simulink model "Falownik_2_4"  (R2023b)
settings: Solver=VariableStepAuto  StartTime=0.0  StopTime=50e-3  FixedStep=1e-9  RelTol=1e-3
libraries: spsSeriesRLCBranchLib x6, spsMosfetLib x4, simulink x2, spsCurrentMeasurementLib x2, spsOnDelayLib x2, spsVoltageMeasurementLib x2, spsDCVoltageSourceLib x1, spsRMSLib x1, spspowerguiLib x1
settings Model: Creator=szymo  LastModifiedBy=rolni
settings OptimizationCC: ReuseModelBlockBuffer=off
settings ModelReferenceCC: EnableRefExpFcnMdlSchedulingChecks=on

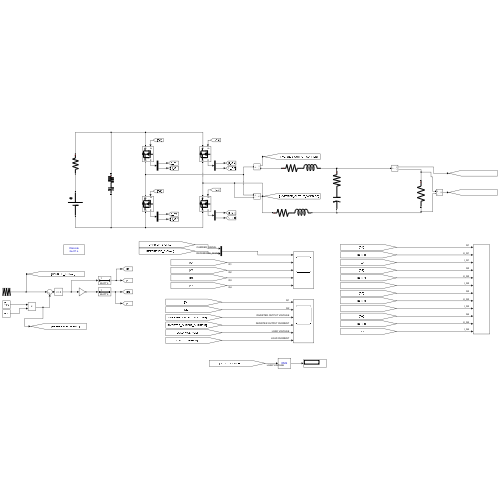
[thumbnail: Simulink's stored preview of the top-level diagram]
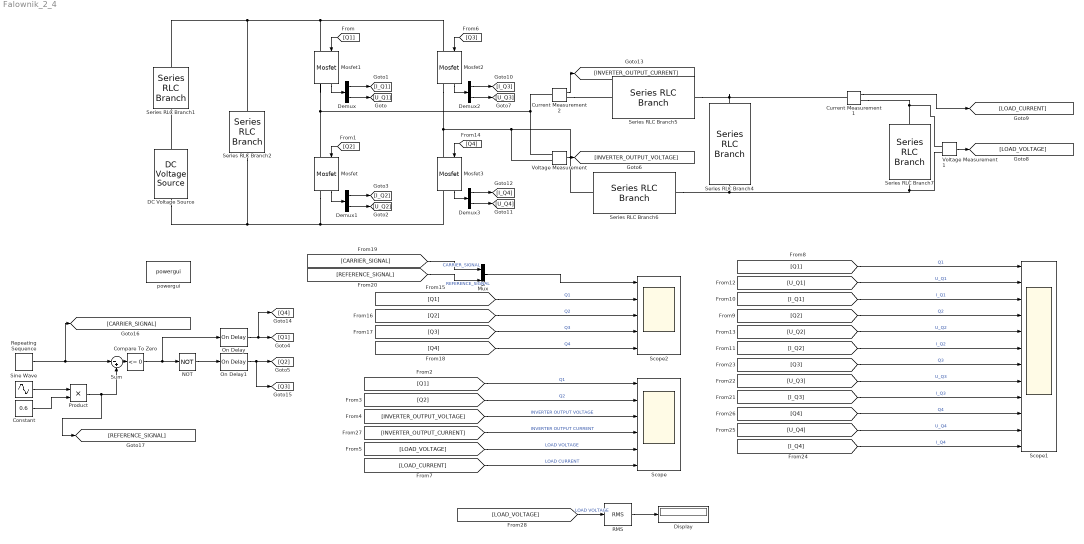
== system Falownik_2_4 ==
  Compare To Zero : simulink/Logic and Bit Operations/Compare To Zero  relop=<=  OutDataTypeStr=boolean
  Constant : Constant  Value=0.6
  Current Measurement1 : spsCurrentMeasurementLib/Current Measurement  PhasorSimulation=off  OutputType=Complex  PSBequivalent=0
  Current Measurement2 : spsCurrentMeasurementLib/Current Measurement  PhasorSimulation=off  OutputType=Complex  PSBequivalent=0
  DC Voltage Source : spsDCVoltageSourceLib/DC Voltage Source  Amplitude=48  Measurements=None
  Demux{,1..3} (4 alike) : Demux  Outputs=2
  Display : Display
  Mosfet{,1..3} (4 alike) : spsMosfetLib/Mosfet  Ron=20e-3  Lon=0  Rd=40e-3  Vfd=1  IC=0  Rs=1e5  Cs=inf  Measurements=on
  Mux : Mux  Inputs=2
  NOT : Logic  Operator=NOT  IconShape=distinctive  AllPortsSameDT=off  OutDataTypeStr=boolean
  On Delay : spsOnDelayLib/On Delay  DelayType=On delay  delay=200e-9  ic=0  Ts=0
  On Delay1 : spsOnDelayLib/On Delay  DelayType=On delay  delay=200e-9  ic=0  Ts=0
  Product : Product
  RMS : spsRMSLib/RMS  TrueRMS=on  Freq=60  RMSInit=120  Ts=0
  Repeating Sequence : simulink/Sources/Repeating Sequence  rep_seq_t=[0 0.5/10e3 1/10e3]  rep_seq_y=[-1 1 -1]
  Scope : Scope  NumInputPorts=6
  Scope1 : Scope  NumInputPorts=12
  Scope2 : Scope  NumInputPorts=5
  Series RLC Branch1 : spsSeriesRLCBranchLib/Series RLC Branch  LConnTagsString=__new0  RConnTagsString=__new0  BranchType=R  Resistance=100e-3  Inductance=1e-3  SetiL0=off  InitialCurrent=0  Capacitance=1e-3  Setx0=on  InitialVoltage=400  Measurements=None
  Series RLC Branch2 : spsSeriesRLCBranchLib/Series RLC Branch  LConnTagsString=__new0  RConnTagsString=__new0  BranchType=RC  Resistance=100e-3  Inductance=1e-3  SetiL0=off  InitialCurrent=0  Capacitance=1e-3  Setx0=on  InitialVoltage=48  Measurements=None
  Series RLC Branch4 : spsSeriesRLCBranchLib/Series RLC Branch  LConnTagsString=__new0  RConnTagsString=__new0  BranchType=RC  Resistance=5e-3  Inductance=4e-6  SetiL0=off  InitialCurrent=0  Capacitance=15e-6  Setx0=off  InitialVoltage=200  Measurements=None
  Series RLC Branch5 : spsSeriesRLCBranchLib/Series RLC Branch  LConnTagsString=__new0  RConnTagsString=__new0  BranchType=RL  Resistance=30e-3  Inductance=147e-6  SetiL0=off  InitialCurrent=0  Capacitance=470e-6  Setx0=on  InitialVoltage=200  Measurements=None
  Series RLC Branch6 : spsSeriesRLCBranchLib/Series RLC Branch  LConnTagsString=__new0  RConnTagsString=__new0  BranchType=RL  Resistance=30e-3  Inductance=147e-6  SetiL0=off  InitialCurrent=0  Capacitance=470e-6  Setx0=on  InitialVoltage=200  Measurements=None
  Series RLC Branch7 : spsSeriesRLCBranchLib/Series RLC Branch  LConnTagsString=__new0  RConnTagsString=__new0  BranchType=R  Resistance=7.7  Inductance=1e-3  SetiL0=off  InitialCurrent=0  Capacitance=470e-6  Setx0=on  InitialVoltage=200  Measurements=None
  Sine Wave : Sin  Frequency=314.16  SampleTime=0
  Sum : Sum  Inputs=|-+
  Voltage Measurement : spsVoltageMeasurementLib/Voltage Measurement  PhasorSimulation=off  OutputType=Complex  PSBequivalent=0
  Voltage Measurement1 : spsVoltageMeasurementLib/Voltage Measurement  PhasorSimulation=off  OutputType=Complex  PSBequivalent=0
  powergui : spspowerguiLib/powergui  Priority=1  SimulationMode=Discrete  SampleTime=200e-9  frequency=60  Iterations=50  frequencyindice=0  Pbase=100e6  ErrMax=1e-4  UnitsV=kV  UnitsW=MW  buscounter=0  FunctionMessages=off  echomessages=off  EnableUseOfTLC=off  CurrentSourceSwitches=off  DisableSnubberDevices=off  DisableRonSwitches=off  DisableVfSwitches=off  DisplayEquations=off  AutomaticDiscreteSolvers=off  SolverType=Tustin/Backward Euler (TBE)  Interpol=off  ExternalGateDelay=off  methode=off  Ts=100  x0status=blocks  SPID=on  SwTol=0  HookPort=off  NonlinearTolerance=1e-4  nMaxIteration=100  ContinueOnMaxIteration=off  RestoreLinks=warning  ResistiveCurrentMeasurement=off  Frange=[0:2:500]  Ylog=off  Xlog=on  ShowGrid=off  save=off  variable=ZData  structure=0  ZoomFFT=off  StartTime=0.0  cycles=1  DisplayStyle=1  fundamental=60  FreqAxis=off  MaxFrequency=1000  frequencyindicesteady=1  RmsSteady=1  display=off
  wires:
  [Q1] -> Mosfet1/1
  [Q2] -> Mosfet/1
  Mosfet1/1 -> Demux/1
  Mosfet/1 -> Demux1/1
  Compare To Zero/1 -> On Delay/1, NOT/1
  NOT/1 -> On Delay1/1
  On Delay/1 -> [Q4], [Q1]
  On Delay1/1 -> [Q3], [Q2]
  [Q1] -> Scope/1  "Q1"
  [Q2] -> Scope/2  "Q2"
  [INVERTER_OUTPUT_VOLTAGE] -> Scope/3  "INVERTER OUTPUT VOLTAGE"
  [LOAD_VOLTAGE] -> Scope/5  "LOAD VOLTAGE"
  [LOAD_CURRENT] -> Scope/6  "LOAD CURRENT"
  [Q2] -> Scope1/4  "Q2"
  [U_Q1] -> Scope1/2  "U_Q1"
  [I_Q1] -> Scope1/3  "I_Q1"
  [U_Q2] -> Scope1/5  "U_Q2"
  [I_Q2] -> Scope1/6  "I_Q2"
  [Q1] -> Scope1/1  "Q1"
  Voltage Measurement/1 -> [INVERTER_OUTPUT_VOLTAGE]
  Voltage Measurement1/1 -> [LOAD_VOLTAGE]
  Current Measurement1/1 -> [LOAD_CURRENT]
  Demux1/1 -> [I_Q2]
  Demux1/2 -> [U_Q2]
  Demux/2 -> [U_Q1]
  Demux/1 -> [I_Q1]
  Demux2/2 -> [U_Q3]
  Mosfet2/1 -> Demux2/1
  [Q3] -> Mosfet2/1
  Demux2/1 -> [I_Q3]
  Demux3/2 -> [U_Q4]
  Mosfet3/1 -> Demux3/1
  [Q4] -> Mosfet3/1
  Demux3/1 -> [I_Q4]
  Current Measurement2/1 -> [INVERTER_OUTPUT_CURRENT]
  Sum/1 -> Compare To Zero/1
  Sine Wave/1 -> Product/1
  Constant/1 -> Product/2
  Product/1 -> [REFERENCE_SIGNAL], Sum/2
  Repeating Sequence/1 -> [CARRIER_SIGNAL], Sum/1
  [Q4] -> Scope2/5  "Q4"
  [Q3] -> Scope2/4  "Q3"
  Mux/1 -> Scope2/1
  [Q1] -> Scope2/2  "Q1"
  [Q2] -> Scope2/3  "Q2"
  [REFERENCE_SIGNAL] -> Mux/2  "REFERENCE_SIGNAL"
  [CARRIER_SIGNAL] -> Mux/1  "CARRIER_SIGNAL"
  [U_Q3] -> Scope1/8  "U_Q3"
  [Q3] -> Scope1/7  "Q3"
  [I_Q3] -> Scope1/9  "I_Q3"
  [U_Q4] -> Scope1/11  "U_Q4"
  [Q4] -> Scope1/10  "Q4"
  [I_Q4] -> Scope1/12  "I_Q4"
  [INVERTER_OUTPUT_CURRENT] -> Scope/4  "INVERTER OUTPUT CURRENT"
  [LOAD_VOLTAGE] -> RMS/1  "LOAD VOLTAGE"
  RMS/1 -> Display/1
  connections:
  Mosfet1/RConn1 -- Voltage Measurement/LConn1 -- Current Measurement2/LConn1 -- Mosfet/LConn1
  DC Voltage Source/RConn1 -- Series RLC Branch1/RConn1
  Mosfet2/RConn1 -- Voltage Measurement/LConn2 -- Series RLC Branch6/LConn1 -- Mosfet3/LConn1
  Current Measurement1/RConn1 -- Series RLC Branch7/LConn1 -- Voltage Measurement1/LConn1
  Series RLC Branch1/LConn1 -- Series RLC Branch2/LConn1 -- Mosfet1/LConn1 -- Mosfet2/LConn1
  DC Voltage Source/LConn1 -- Series RLC Branch2/RConn1 -- Mosfet3/RConn1 -- Mosfet/RConn1
  Current Measurement2/RConn1 -- Series RLC Branch5/LConn1
  Series RLC Branch5/RConn1 -- Current Measurement1/LConn1 -- Series RLC Branch4/LConn1
  Series RLC Branch6/RConn1 -- Series RLC Branch4/RConn1 -- Voltage Measurement1/LConn2 -- Series RLC Branch7/RConn1
